simulink library "INT_PTOEnblSwt_DD"  (R2016b)
settings: Solver=VariableStepAuto  StartTime=0.0  StopTime=10.0  RelTol=1e-3
settings Model: Creator=bianxuyin  LastModifiedBy=bianxuyin

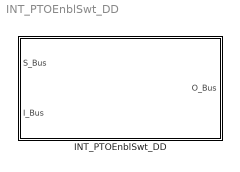
== system INT_PTOEnblSwt_DD ==
  INT_PTOEnblSwt_DD : Subsystem

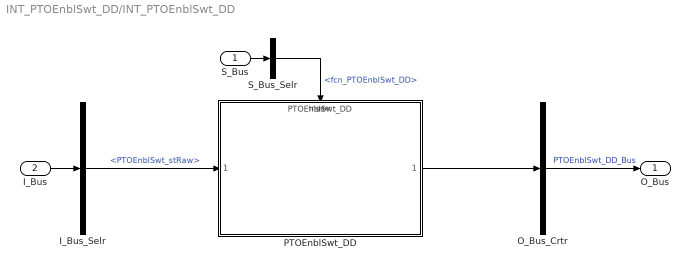
== system INT_PTOEnblSwt_DD/INT_PTOEnblSwt_DD ==
  S_Bus : Inport
  I_Bus : Inport  Port=2
  I_Bus_Selr : BusSelector  OutputSignals=PTOEnblSwt_stRaw
  O_Bus_Crtr : BusCreator  Inputs=1
  PTOEnblSwt_DD : ModelReference  ModelNameDialog=PTOEnblSwt_DD  SimulationMode=Normal  ModelReferenceVersion=1.4  TriggerPortName=function  TriggerPortTriggerType=function-call  TriggerPortStatesWhenEnabling=held
  S_Bus_Selr : BusSelector  OutputSignals=fcn_PTOEnblSwt_DD
  O_Bus : Outport
  wires:
  S_Bus_Selr/1 -> PTOEnblSwt_DD/Trigger  "<fcn_PTOEnblSwt_DD>"
  S_Bus/1 -> S_Bus_Selr/1
  I_Bus/1 -> I_Bus_Selr/1
  I_Bus_Selr/1 -> PTOEnblSwt_DD/1  "<PTOEnblSwt_stRaw>"
  O_Bus_Crtr/1 -> O_Bus/1  "PTOEnblSwt_DD_Bus"
  PTOEnblSwt_DD/1 -> O_Bus_Crtr/1
